simulink model "CalorieController"  (R2024b)
settings: Solver=VariableStepAuto  StartTime=0.0  StopTime=2000  RelTol=1e-3
libraries: cstblocks x1
settings Model: Creator=TC63  LastModifiedBy=TC63

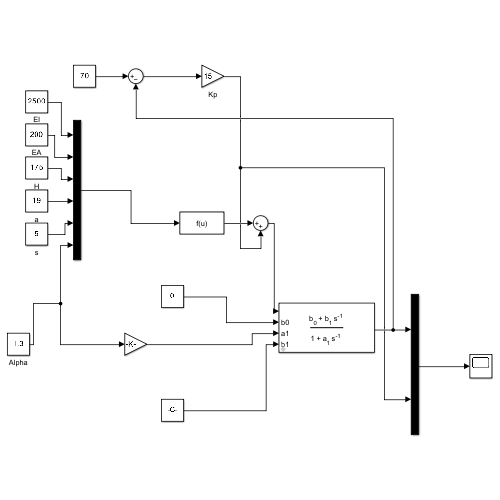
[thumbnail: Simulink's stored preview of the top-level diagram]
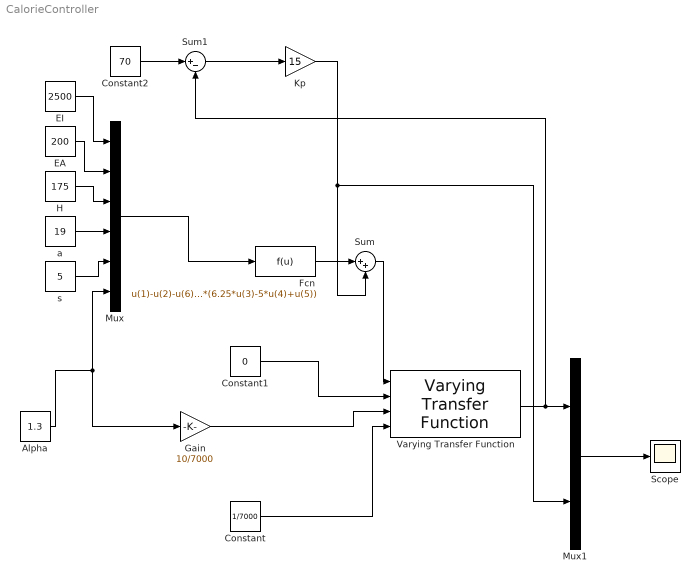
== system CalorieController ==
  Alpha : Constant  Value=1.3
  Constant : Constant  Value=1/7000
  Constant1 : Constant  Value=0
  Constant2 : Constant  Value=70
  EA : Constant  Value=200
  EI : Constant  Value=2500
  Fcn : Fcn  Expr=u(1)-u(2)-u(6)*(6.25*u(3)-5*u(4)+u(5))
  Gain : Gain  Gain=10/7000
  H : Constant  Value=175
  Kp : Gain  Gain=15
  Mux : Mux  Inputs=6
  Mux1 : Mux  Inputs=2
  Scope : Scope
  Sum : Sum  Inputs=|++
  Sum1 : Sum  Inputs=|+-
  Varying Transfer Function : cstblocks/Linear Parameter Varying/Varying Transfer Function  N=1  Feedthrough=on
      link override Integrator1: InitialCondition=65.5
  a : Constant  Value=19
  s : Constant  Value=5
  wires:
  Gain/1 -> Varying Transfer Function/3
  Alpha/1 -> Gain/1, Mux/6
  Constant/1 -> Varying Transfer Function/4
  Constant1/1 -> Varying Transfer Function/2
  EI/1 -> Mux/1
  EA/1 -> Mux/2
  Mux/1 -> Fcn/1
  H/1 -> Mux/3
  a/1 -> Mux/4
  s/1 -> Mux/5
  Varying Transfer Function/1 -> Sum1/2, Mux1/1
  Mux1/1 -> Scope/1
  Fcn/1 -> Sum/1
  Constant2/1 -> Sum1/1
  Sum1/1 -> Kp/1
  Sum/1 -> Varying Transfer Function/1
  Kp/1 -> Mux1/2, Sum/2
